simulink model "DOO_test"  (R2020a)
settings: Solver=FixedStepAuto  StartTime=0.0  StopTime=10.0  FixedStep=1e-3  RelTol=1e-3  EnableMultiTasking=on
settings Model: ExtModeTrigDuration=5  Creator=zhanz173  LastModifiedBy=zhanz173
settings OptimizationCC: EnhancedBackFolding=on  PassReuseOutputArgsAs=Individual arguments  ZeroExternalMemoryAtStartup=off  ZeroInternalMemoryAtStartup=off  MaxStackSize=64  OptimizeBlockOrder=speed  DifferentSizesBufferReuse=on  OptimizationCustomize=off  EfficientTunableParamExpr=on
settings DebuggingCC: ParameterTunabilityLossMsg=error
settings HardwareCC: ProdBitPerPointer=32  ProdBitPerSizeT=32  ProdBitPerPtrDiffT=32  ProdLargestAtomicInteger=Long  ProdLargestAtomicFloat=Double  ProdWordSize=32  ProdHWDeviceType=ARM Compatible->ARM Cortex  TargetBitPerPointer=64  TargetBitPerSizeT=64  TargetBitPerPtrDiffT=64  TargetLongLongMode=on  TargetIntDivRoundTo=Zero  TargetEndianess=LittleEndian  TargetWordSize=64  TargetHWDeviceType=Custom Processor->MATLAB Host Computer  ProdEqTarget=off
settings SFSimCC: MATLABDynamicMemAlloc=off
settings RTWCC: SystemTargetFile=ert.tlc  HardwareBoard=NXP FRDM-K64F  TemplateMakefile=ert_default_tmf  Toolchain=GNU Tools for ARM Embedded Processors
settings CodeAppCC: ForceParamTrailComments=on  IgnoreCustomStorageClasses=off  OperatorAnnotations=on  SimulinkDataObjDesc=on  SFDataObjDesc=on  InsertBlockDesc=on

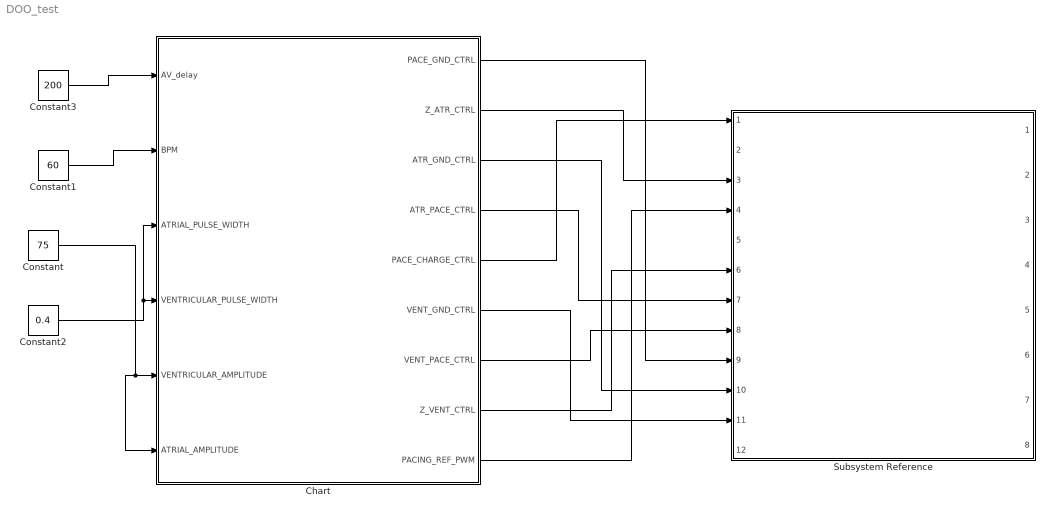
== system DOO_test ==
  Chart : Stateflow chart  TreatAsAtomicUnit=on
  Constant : Constant  Value=75
  Constant1 : Constant  Value=60
  Constant2 : Constant  Value=0.4
  Constant3 : Constant  Value=200
  Subsystem Reference : Subsystem  ReferencedSubsystem=k64f_subsystem
  wires:
  Constant/1 -> Chart/6(ATRIAL_AMPLITUDE), Chart/5(VENTRICULAR_AMPLITUDE)
  Constant2/1 -> Chart/3(ATRIAL_PULSE_WIDTH), Chart/4(VENTRICULAR_PULSE_WIDTH)
  Constant1/1 -> Chart/2(BPM)
  Constant3/1 -> Chart/1(AV_delay)
  Chart/1(PACE_GND_CTRL) -> Subsystem Reference/9
  Chart/2(Z_ATR_CTRL) -> Subsystem Reference/3
  Chart/3(ATR_GND_CTRL) -> Subsystem Reference/10
  Chart/4(ATR_PACE_CTRL) -> Subsystem Reference/7
  Chart/6(VENT_GND_CTRL) -> Subsystem Reference/11
  Chart/8(Z_VENT_CTRL) -> Subsystem Reference/6
  Chart/9(PACING_REF_PWM) -> Subsystem Reference/4
  Chart/5(PACE_CHARGE_CTRL) -> Subsystem Reference/1
  Chart/7(VENT_PACE_CTRL) -> Subsystem Reference/8

== stateflow chart DOO_test/Chart ==
  note: DOO mode paces the atrium then ventricle at a constant rate regardless of the natural heartbeat
  state PULSE_ATR
    entry:
    PACE_CHARGE_CTRL = 0;
    PACE_GND_CTRL = 1;
    VENT_GND_CTRL = 0;
    VENT_PACE_CTRL = 0;
    Z_ATR_CTRL = 0;
    Z_VENT_CTRL = 0;
    ATR_GND_CTRL = 0;
    ATR_PACE_CTRL = 1;
  state CHARGE
    entry:
    ATR_PACE_CTRL = 0;
    VENT_PACE_CTRL = 0;
    PACING_REF_PWM = ATRIAL_AMPLITUDE;
    PACE_CHARGE_CTRL = 1;
  state DISCHARGE
    entry:
    PACE_GND_CTRL = 1;
    VENT_PACE_CTRL = 0;
    Z_ATR_CTRL = 0;
    Z_VENT_CTRL = 0;
    ATR_PACE_CTRL = 0;
    ATR_GND_CTRL = 1;
    VENT_GND_CTRL = 0;
  state CHARGE1
    entry:
    ATR_PACE_CTRL = 0;
    VENT_PACE_CTRL = 0;
    PACING_REF_PWM = VENTRICULAR_AMPLITUDE;
    PACE_CHARGE_CTRL = 1;
  state PULSE_VENT
    entry:
    PACE_CHARGE_CTRL = 0;
    PACE_GND_CTRL = 1;
    ATR_PACE_CTRL = 0;
    ATR_GND_CTRL = 0;
    Z_ATR_CTRL = 0;
    Z_VENT_CTRL = 0;
    VENT_GND_CTRL = 0;
    VENT_PACE_CTRL = 1;
  state DISCHARGE1
    entry:
    PACE_GND_CTRL = 1;
    VENT_PACE_CTRL = 0;
    Z_ATR_CTRL = 0;
    Z_VENT_CTRL = 0;
    ATR_PACE_CTRL = 0;
    ATR_GND_CTRL = 0;
    VENT_GND_CTRL = 1;
  (default) -> CHARGE
  CHARGE -> PULSE_ATR : after(60/BPM*1000 - AV_delay, msec)
  DISCHARGE1 -> CHARGE
  PULSE_ATR -> DISCHARGE : after(ATRIAL_PULSE_WIDTH, msec)
  DISCHARGE -> CHARGE1
  CHARGE1 -> PULSE_VENT : after(AV_delay,msec)
  PULSE_VENT -> DISCHARGE1 : after(VENTRICULAR_PULSE_WIDTH, msec)
  data: PACE_GND_CTRL output; Z_ATR_CTRL output; AV_delay input; BPM input; ATR_GND_CTRL output; ATR_PACE_CTRL output; PACE_CHARGE_CTRL output; VENT_GND_CTRL output; VENT_PACE_CTRL output; Z_VENT_CTRL output; ATRIAL_PULSE_WIDTH input; VENTRICULAR_PULSE_WIDTH input; VENTRICULAR_AMPLITUDE input; ATRIAL_AMPLITUDE input; PACING_REF_PWM output
